simulink model "nar_test"  (Simulink 7.8)
settings: Solver=ode45  StartTime=0.0  StopTime=5000  RelTol=1e-3
undefined symbols (not defined in the file or in its folder): pfb_coeff_gen_calc
libraries: xbsIndex_r4 x1069, casper_library_misc x63, xps_library x35, casper_library_delays x19, xbsReplacements_r4 x10, gavrt_library x4, simulink x1
(part 1 of 14)
settings Model: Creator=dan  LastModifiedBy=dan
settings Model: ModifiedComment=|
  | dan -- Sun Apr 07 12:16:58 2013 -- Version 1.75
  | 
  | Added in an always on snap (not through demux)
settings Model: ModifiedHistory=|
  | dan -- Sun Apr 07 12:16:58 2013 -- Version 1.75
  | 
  | Added in an always on snap (not through demux)
  | 
  | dan -- Sat Apr 06 15:53:26 2013 -- Version 1.74
  | 
  | Added accumulation counter to NAR
  | Removed on-off snap blocks, as I think they're not needed
  | 
  | dan -- Fri Apr 05 00:58:20 2013 -- Version 1.73
  | 
  | Fixed pcore issue
  | 
  | dan -- Fri Apr 05 00:24:31 2013 -- Version 1.72
  | Switched over to blackboxed ISE 11.1 generated FFT
  | 
  | dan -- Fri Apr 05 00:21:17 2013 -- Version 1.71
  | 
  | Trying a really really old FFT from 11.1, blackboxed
  | 
  | dan -- Fri Apr 05 00:21:00 2013 -- Version 1.70
  | 
  | 
  | dan -- Thu Apr 04 16:23:17 2013 -- Version 1.69
  | 
  | Added delay back to just before nar snap blocks, as  sync appears to be triggered later with new FFT
  | 
  | dan -- Thu Apr 04 15:15:10 2013 -- Version 1.68
  | 
  | Compiled OK, now testing design
  | 
  | dan -- Thu Apr 04 14:31:56 2013 -- Version 1.67
  | 
  | Black boxed the NAR 32 point FFTs, which were generated using 'simulink13' on phaezar. This is to try and resolve FFT issues (output seems to be garbage).
  | 
  | dan -- Wed Apr 03 15:57:11 2013 -- Version 1.66
  | 
  | quant snap now triggered by sync signal
  | 
  | dan -- Wed Apr 03 15:52:39 2013 -- Version 1.65
  | 
  | 
  | dan -- Wed Apr 03 12:50:37 2013 -- Version 1.64
  | changed delay_bram on ad c snapso that it now delays by 1/4 less (as ADC samples are 4x FPGA clock)
  | 
  | dan -- Wed Apr 03 11:56:50 2013 -- Version 1.63
  | increased size of adc snap blocks
  | 
  | dan -- Tue Apr 02 22:16:52 2013 -- Version 1.62
  | fixed mislabelled snap_cal_x and snap_cal_y
  | 
  | dan -- Tue Apr 02 21:19:46 2013 -- Version 1.61
  | 
  | ADC snap now delays by 8192
  | trying to fix dc offset in nar output
  | 
  | dan -- Tue Apr 02 19:54:07 2013 -- Version 1.60
  | 
  | Changed snap block names in NAR block
  | 
  | dan -- Mon Apr 01 17:00:32 2013 -- Version 1.59
  | 
  | Test rig for nar block. Inverted logic in NAR demux block (it was the wrong way round)

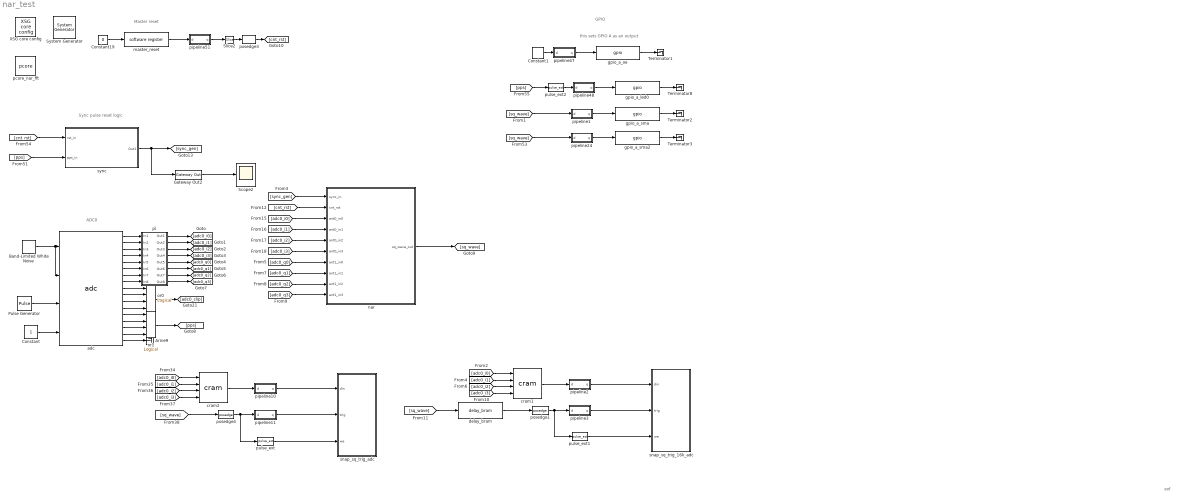
== system nar_test ==
  note: ADC0
  note: Sync pulse reset logic
  note: Master reset
  note: this sets GPIO A as an output
  note: GPIO
  note: eof
  " System Generator" : xbsIndex_r4/ System Generator  Tag=genX  xilinxfamily=virtex5  part=xc5vsx95t  speed=-1  package=ff1136  synthesis_tool=XST  clock_wrapper=Clock Enables  directory=./noise_diode13_bb_11x/sysgen  proj_type=Project Navigator  Synth_file=XST Defaults  Impl_file=ISE Defaults  testbench=off  simulink_period=1  sysclk_period=5  dcm_input_clock_period=100  incr_netlist=off  trim_vbits=Everywhere in SubSystem  dbl_ovrd=According to Block Masks  core_generation=According to Block Masks  run_coregen=off  deprecated_control=off  eval_field=0  block_type=sysgen
  Arnie9 : Terminator
  Band-Limited White Noise : simulink/Sources/Band-Limited White Noise  Cov=[0.1]  Ts=0.1  seed=[23341]
  Constant : Constant
  Constant1 : xbsIndex_r4/Constant  const=0  gui_display_data_type=Boolean  arith_type=Boolean  n_bits=16  bin_pt=14  preci_type=Single  exp_width=8  frac_width=24  explicit_period=on  period=1  equ=P=C  opselect=C  inp2=PCIN>>17  opr=+  inp1=P  carry=CIN  dbl_ovrd=off  block_type=constant
  Constant19 : Constant  Value=0
  Gateway Out2 : xbsIndex_r4/Gateway Out  inherit_from_input=off  hdl_port=on  timing_constraint=None  locs_specified=off  LOCs={}  UseAsDAC=off  DACChannel='1'  block_type=gatewayout
      settings: infoedit="Gateway out block.  Converts Xilinx fixed-point or floating-point type inputs into ouputs of type Simulink integer, single, double, or fixed point.<br><br>Hardware notes:  In hardware these blocks become top level output ports or are discarded, depending on how they are configured."
  Pulse Generator : DiscretePulseGenerator  PulseType=Time based  Period=2^27  PulseWidth=1/2^27
  Scope2 : Scope
  Slice2 : xbsIndex_r4/Slice  nbits=1  boolean_output=on  mode=Lower Bit Location + Width  bit1=0  base1=MSB of Input  bit0=0  base0=LSB of Input  dbl_ovrd=off  block_type=slice
      settings: infoedit="Extracts a given range of bits from each input sample and presents it at the output.  The output type is ordinarily unsigned with binary point at zero, but can be Boolean when the slice is one bit wide.<P><P>Hardware notes: In hardware this block costs nothing."  block_version=10.1.3
  Terminator{1..3,8} (4 alike) : Terminator
  XSG core config : xps_library/XSG core config  Tag=xps:xsg  hw_sys=ROACH:sx95t  ibob_linux=off  clk_src=adc0_clk  iBOB_clk_src=sys_clk  BEE2_ctrl_clk_src=sys_clk  BEE2_usr_clk_src=sys_clk  ROACH_clk_src=adc0_clk  ROACH2_clk_src=adc0_clk  CORR_clk_src=sys_clk  gpio_clk_io_group=iBOB:sma  gpio_clk_bit_index=0  clk_rate=200  sample_period=1  synthesis_tool=XST  mpc_type=powerpc440_ext
  adc : xps_library/adc  Tag=xps:adc  adc_brd=adc0  adc_clk_rate=800  adc_interleave=off  sample_period=1
  cram1 : gavrt_library/cram  num_slice=4
  cram2 : gavrt_library/cram  num_slice=4
  delay_bram : casper_library_delays/delay_bram  DelayLen=2^13/4  bram_latency=4  use_dsp48=off
  gpio_a_led0 : xps_library/gpio  Tag=xps:gpio  io_group=ROACH:gpioa  io_dir=out  arith_type=Boolean  bitwidth=1  bin_pt=0  bit_index=4  sample_period=1  use_single_ended=off  use_ddr=off  reg_iob=on  reg_clk_phase=0  termination=None
  gpio_a_oe : xps_library/gpio  Tag=xps:gpio  io_group=ROACH:gpioa_oe_n  io_dir=out  arith_type=Boolean  bitwidth=1  bin_pt=0  bit_index=0  sample_period=1  use_single_ended=off  use_ddr=off  reg_iob=on  reg_clk_phase=0  termination=None
  gpio_a_sma : xps_library/gpio  Tag=xps:gpio  io_group=ROACH:gpioa  io_dir=out  arith_type=Boolean  bitwidth=1  bin_pt=0  bit_index=6  sample_period=1  use_single_ended=off  use_ddr=off  reg_iob=on  reg_clk_phase=0  termination=Pulldown
  gpio_a_sma2 : xps_library/gpio  Tag=xps:gpio  io_group=ROACH:gpioa  io_dir=out  arith_type=Boolean  bitwidth=1  bin_pt=0  bit_index=7  sample_period=1  use_single_ended=off  use_ddr=off  reg_iob=on  reg_clk_phase=0  termination=Pullup
  master_reset : xps_library/software register  Tag=xps:sw_reg  io_dir=From Processor  arith_type=Unsigned  bitwidth=32  bin_pt=0  sample_period=1  gw_name=nar_test_master_reset_user_data_out
      link override coarse_r01_cnt_rst_user_data_out: arith_type=Unsigned  n_bits=32  bin_pt=0  period=1
      link override coarse_r02_cnt_rst_user_data_out: arith_type=Unsigned  n_bits=32  bin_pt=0  period=1
      link override coarse_r03_cnt_rst_user_data_out: arith_type=Unsigned  n_bits=32  bin_pt=0  period=1
      link override coarse_r04_cnt_rst_user_data_out: arith_type=Unsigned  n_bits=32  bin_pt=0  period=1
      link override coarse_r06_cnt_rst_user_data_out: arith_type=Unsigned  n_bits=32  bin_pt=0  period=1
      link override coarse_r07_cnt_rst_user_data_out: arith_type=Unsigned  n_bits=32  bin_pt=0  period=1
      link override coarse_r08_cnt_rst_user_data_out: arith_type=Unsigned  n_bits=32  bin_pt=0  period=1
      link override coarse_r09_cnt_rst_user_data_out: arith_type=Unsigned  n_bits=32  bin_pt=0  period=1
      link override coarse_r10_cnt_rst_user_data_out: arith_type=Unsigned  n_bits=32  bin_pt=0  period=1
      link override coarse_r12_cnt_rst_user_data_out: arith_type=Unsigned  n_bits=32  bin_pt=0  period=1
      link override convert: arith_type=Unsigned  n_bits=32  bin_pt=0
      link override qdr_single_r01_cnt_rst_user_data_out: arith_type=Unsigned  n_bits=32  bin_pt=0  period=1
      link override qdr_single_r02_cnt_rst_user_data_out: arith_type=Unsigned  n_bits=32  bin_pt=0  period=1
      link override qdr_single_r04_cnt_rst_user_data_out: arith_type=Unsigned  n_bits=32  bin_pt=0  period=1
      link override r_spec_2048_r102_cnt_rst_user_data_out: arith_type=Unsigned  n_bits=32  bin_pt=0  period=1
      link override r_spec_2048_r102_nosim_cnt_rst_user_data_out: arith_type=Unsigned  n_bits=32  bin_pt=0  period=1
      link override r_spec_2048_r103_cnt_rst_user_data_out: arith_type=Unsigned  n_bits=32  bin_pt=0  period=1
      link override r_spec_2048_r104_cnt_rst_user_data_out: arith_type=Unsigned  n_bits=32  bin_pt=0  period=1
      link override r_spec_2048_r104_test0_cnt_rst_user_data_out: arith_type=Unsigned  n_bits=32  bin_pt=0  period=1
      link override r_spec_2048_r104_test_cnt_rst_user_data_out: arith_type=Unsigned  n_bits=32  bin_pt=0  period=1
      link override r_spec_2048_r105_cnt_rst_user_data_out: arith_type=Unsigned  n_bits=32  bin_pt=0  period=1
      link override r_spec_test0_cnt_rst_user_data_out: arith_type=Unsigned  n_bits=32  bin_pt=0  period=1
      link override r_spec_test4_cnt_rst_user_data_out: arith_type=Unsigned  n_bits=32  bin_pt=0  period=1
      link override roach_spec_no10gbe_sync_cnt_rst_user_data_out: arith_type=Unsigned  n_bits=32  bin_pt=0  period=1
      link override roach_spec_rst_cnt_user_data_out: arith_type=Unsigned  n_bits=32  bin_pt=0  period=1
      link override roach_spec_rst_sync_cnt_user_data_out: arith_type=Unsigned  n_bits=32  bin_pt=0  period=1
      link override toast_256ch_16bit_r02_cnt_rst_user_data_out: arith_type=Unsigned  n_bits=32  bin_pt=0  period=1
      link override toast_256ch_16bit_r04_cnt_rst_user_data_out: arith_type=Unsigned  n_bits=32  bin_pt=0  period=1
      link override toast_256ch_16bit_r05_cnt_rst_user_data_out: arith_type=Unsigned  n_bits=32  bin_pt=0  period=1
  nar : Subsystem
  or0 : xbsIndex_r4/Logical  logical_function=OR  inputs=4  en=off  latency=2  precision=Full  arith_type=Unsigned  n_bits=16  bin_pt=0  align_bp=off  dbl_ovrd=off  block_type=logical
  or1 : xbsIndex_r4/Logical  logical_function=OR  inputs=4  en=off  latency=2  precision=Full  arith_type=Unsigned  n_bits=16  bin_pt=0  align_bp=off  dbl_ovrd=off  block_type=logical
  pcore_nar_fft : xps_library/pcore  Tag=xps:pcore  pcore_path=./bb/fft_32pt_11x_core/fft_32pt_11x_core.ngc
  pipeline1 : Subsystem  AncestorBlock=casper_library_delays/pipeline  mask(pipeline){latency=1}
      mask help:
      | An explicitly laid-out delay line to avoid mapping to SRL16s
      | for use in pipelining to help achieve timing closure.
      mask init:
      | pipeline_init(gcb,'latency',latency);
      settings: AttributesFormatString=Latency = %<latency>
      mask Display:
      | port_label('input', 1, 'd');
      | port_label('output', 1, 'q');
      | disp(['Z^-', num2str(latency)]);
  pipeline10 : Subsystem  AncestorBlock=casper_library_delays/pipeline  mask(pipeline){latency=1}
      mask help:
      | An explicitly laid-out delay line to avoid mapping to SRL16s
      | for use in pipelining to help achieve timing closure.
      mask init:
      | pipeline_init(gcb,'latency',latency);
      settings: AttributesFormatString=Latency = %<latency>
      mask Display:
      | port_label('input', 1, 'd');
      | port_label('output', 1, 'q');
      | disp(['Z^-', num2str(latency)]);
  pipeline11 : Subsystem  AncestorBlock=casper_library_delays/pipeline  mask(pipeline){latency=1}
      mask help:
      | An explicitly laid-out delay line to avoid mapping to SRL16s
      | for use in pipelining to help achieve timing closure.
      mask init:
      | pipeline_init(gcb,'latency',latency);
      settings: AttributesFormatString=Latency = %<latency>
      mask Display:
      | port_label('input', 1, 'd');
      | port_label('output', 1, 'q');
      | disp(['Z^-', num2str(latency)]);
  pipeline2 : Subsystem  AncestorBlock=casper_library_delays/pipeline  mask(pipeline){latency=1}
      mask help:
      | An explicitly laid-out delay line to avoid mapping to SRL16s
      | for use in pipelining to help achieve timing closure.
      mask init:
      | pipeline_init(gcb,'latency',latency);
      settings: AttributesFormatString=Latency = %<latency>
      mask Display:
      | port_label('input', 1, 'd');
      | port_label('output', 1, 'q');
      | disp(['Z^-', num2str(latency)]);
  pipeline24 : Subsystem  AncestorBlock=casper_library_delays/pipeline  mask(pipeline){latency=1}
      mask help:
      | An explicitly laid-out delay line to avoid mapping to SRL16s
      | for use in pipelining to help achieve timing closure.
      mask init:
      | pipeline_init(gcb,'latency',latency);
      settings: AttributesFormatString=Latency = %<latency>
      mask Display:
      | port_label('input', 1, 'd');
      | port_label('output', 1, 'q');
      | disp(['Z^-', num2str(latency)]);
  pipeline3 : Subsystem  AncestorBlock=casper_library_delays/pipeline  mask(pipeline){latency=1}
      mask help:
      | An explicitly laid-out delay line to avoid mapping to SRL16s
      | for use in pipelining to help achieve timing closure.
      mask init:
      | pipeline_init(gcb,'latency',latency);
      settings: AttributesFormatString=Latency = %<latency>
      mask Display:
      | port_label('input', 1, 'd');
      | port_label('output', 1, 'q');
      | disp(['Z^-', num2str(latency)]);
  pipeline47 : Subsystem  AncestorBlock=casper_library_delays/pipeline  mask(pipeline){latency=1}
      mask help:
      | An explicitly laid-out delay line to avoid mapping to SRL16s
      | for use in pipelining to help achieve timing closure.
      mask init:
      | pipeline_init(gcb,'latency',latency);
      settings: AttributesFormatString=Latency = %<latency>
      mask Display:
      | port_label('input', 1, 'd');
      | port_label('output', 1, 'q');
      | disp(['Z^-', num2str(latency)]);
  pipeline48 : Subsystem  AncestorBlock=casper_library_delays/pipeline  mask(pipeline){latency=1}
      mask help:
      | An explicitly laid-out delay line to avoid mapping to SRL16s
      | for use in pipelining to help achieve timing closure.
      mask init:
      | pipeline_init(gcb,'latency',latency);
      settings: AttributesFormatString=Latency = %<latency>
      mask Display:
      | port_label('input', 1, 'd');
      | port_label('output', 1, 'q');
      | disp(['Z^-', num2str(latency)]);
  pipeline51 : Subsystem  AncestorBlock=casper_library_delays/pipeline  mask(pipeline){latency=1}
      mask help:
      | An explicitly laid-out delay line to avoid mapping to SRL16s
      | for use in pipelining to help achieve timing closure.
      mask init:
      | pipeline_init(gcb,'latency',latency);
      settings: AttributesFormatString=Latency = %<latency>
      mask Display:
      | port_label('input', 1, 'd');
      | port_label('output', 1, 'q');
      | disp(['Z^-', num2str(latency)]);
  pl : Subsystem
  posedge1 : casper_library_misc/posedge  Tag=Rising Edge Detector
  posedge3 : casper_library_misc/posedge  Tag=Rising Edge Detector
  posedge4 : casper_library_misc/posedge  Tag=Rising Edge Detector
  pulse_ext : casper_library_misc/pulse_ext  pulse_len=2^12
  pulse_ext1 : casper_library_misc/pulse_ext  pulse_len=2^12
  pulse_ext2 : casper_library_misc/pulse_ext  pulse_len=2^24
  snap_sq_trig_16k_adc : Subsystem  AncestorBlock=casper_library_scopes/snap  mask(snap){nsamples=13}
      mask prompts: nsamples "No. of samples(2^?)"
      mask help:
      | The <i>snap</i> block provides a packaged solution to capturing data from
      | the FPGA fabric and making it accessible from the CPU.  The block comes in
      | 2 flavors: <i>snap</i> (which captures to a 32 bit wide Shared BRAM), and
      | <i>snap64</i> (which captures to 2x32 bit wide Shared BRAMs to effect a
      | 64 bit capture).
      mask Help: eval('xlWeb(''http://casper.berkeley.edu/wiki/Snap'')')
  snap_sq_trig_adc : Subsystem  AncestorBlock=casper_library_scopes/snap  mask(snap){nsamples=13}
      mask prompts: nsamples "No. of samples(2^?)"
      mask help:
      | The <i>snap</i> block provides a packaged solution to capturing data from
      | the FPGA fabric and making it accessible from the CPU.  The block comes in
      | 2 flavors: <i>snap</i> (which captures to a 32 bit wide Shared BRAM), and
      | <i>snap64</i> (which captures to 2x32 bit wide Shared BRAMs to effect a
      | 64 bit capture).
      mask Help: eval('xlWeb(''http://casper.berkeley.edu/wiki/Snap'')')
  sync : Subsystem  AncestorBlock=hipsr_library/sync
  wires:
  Band-Limited White Noise/1 -> adc/2, adc/1
  Pulse Generator/1 -> adc/3
  Constant/1 -> adc/4
  adc/9 -> or0/1
  adc/10 -> or0/2
  adc/11 -> or0/3
  adc/12 -> or0/4
  adc/13 -> or1/1
  adc/14 -> or1/2
  adc/15 -> or1/3
  adc/16 -> or1/4
  adc/17 -> Arnie9/1
  or0/1 -> [adc0_clip]
  or1/1 -> [pps]
  adc/1 -> pl/1(In1)
  adc/2 -> pl/2(In2)
  adc/3 -> pl/3(In3)
  adc/4 -> pl/4(In4)
  adc/5 -> pl/5(In5)
  adc/6 -> pl/6(In6)
  adc/7 -> pl/7(In7)
  adc/8 -> pl/8(In8)
  pl/1(Out1) -> [adc0_i0]
  pl/2(Out2) -> [adc0_i1]
  pl/3(Out3) -> [adc0_i2]
  pl/4(Out4) -> [adc0_i3]
  pl/5(Out5) -> [adc0_q0]
  pl/6(Out6) -> [adc0_q1]
  pl/7(Out7) -> [adc0_q2]
  pl/8(Out8) -> [adc0_q3]
  [pps] -> sync/2(pps_in)
  sync/1(Out1) -> [sync_gen], Gateway Out2/1
  [cnt_rst] -> sync/1(rst_in)
  master_reset/1 -> pipeline51/1(d)
  Constant19/1 -> master_reset/1
  pipeline51/1(q) -> Slice2/1
  Slice2/1 -> posedge3/1
  posedge3/1 -> [cnt_rst]
  Constant1/1 -> pipeline47/1(d)
  pipeline47/1(q) -> gpio_a_oe/1
  gpio_a_oe/1 -> Terminator1/1
  pipeline48/1(q) -> gpio_a_led0/1
  gpio_a_led0/1 -> Terminator8/1
  [pps] -> pulse_ext2/1
  pulse_ext2/1 -> pipeline48/1(d)
  pipeline1/1(q) -> gpio_a_sma/1
  gpio_a_sma/1 -> Terminator2/1
  [sq_wave] -> pipeline1/1(d)
  Gateway Out2/1 -> Scope2/1
  pipeline24/1(q) -> gpio_a_sma2/1
  gpio_a_sma2/1 -> Terminator3/1
  [sq_wave] -> pipeline24/1(d)
  pipeline10/1(q) -> snap_sq_trig_adc/1(din)
  pipeline11/1(q) -> snap_sq_trig_adc/2(trig)
  [adc0_i0] -> cram2/1
  [adc0_i1] -> cram2/2
  [adc0_i2] -> cram2/3
  [adc0_i3] -> cram2/4
  cram2/1 -> pipeline10/1(d)
  [sq_wave] -> posedge4/1
  posedge4/1 -> pipeline11/1(d), pulse_ext/1
  pulse_ext/1 -> snap_sq_trig_adc/3(we)
  [sync_gen] -> nar/1(sync_in)
  [adc0_i0] -> nar/3(ant0_in0)
  [adc0_i1] -> nar/4(ant0_in1)
  [adc0_i2] -> nar/5(ant0_in2)
  [adc0_i3] -> nar/6(ant0_in3)
  [adc0_q0] -> nar/7(ant1_in0)
  [adc0_q1] -> nar/8(ant1_in1)
  [adc0_q2] -> nar/9(ant1_in2)
  [adc0_q3] -> nar/10(ant1_in3)
  nar/1(sq_wave_out) -> [sq_wave]
  pipeline2/1(q) -> snap_sq_trig_16k_adc/1(din)
  pipeline3/1(q) -> snap_sq_trig_16k_adc/2(trig)
  [adc0_i0] -> cram1/1
  [adc0_i1] -> cram1/2
  [adc0_i2] -> cram1/3
  [adc0_i3] -> cram1/4
  cram1/1 -> pipeline2/1(d)
  [sq_wave] -> delay_bram/1
  posedge1/1 -> pulse_ext1/1, pipeline3/1(d)
  pulse_ext1/1 -> snap_sq_trig_16k_adc/3(we)
  delay_bram/1 -> posedge1/1
  [cnt_rst] -> nar/2(cnt_rst)
